simulink model "gluehofen"  (Simulink 3.00)
settings: Solver=ode45  StartTime=0.0  StopTime=80000  RelTol=1e-3
undefined symbols (not defined in the file): T

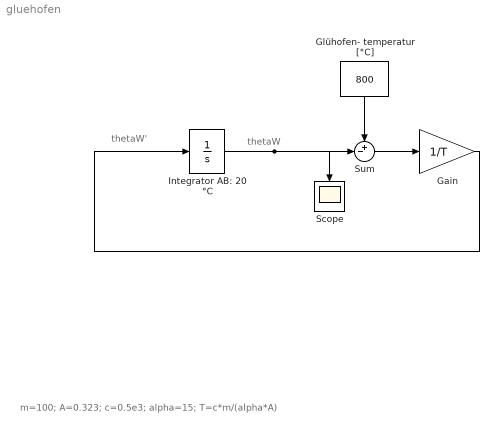
== system gluehofen ==
  note: m=100;
      | A=0.323;
      | c=0.5e3;
      | alpha=15;
      | T=c*m/(alpha*A)
  note: thetaW
  note: thetaW'
  Gain : Gain  Gain=1/T  SaturateOnIntegerOverflow=on
  Glühofen- temperatur [°C] : Constant  Orientation=down  Value=800
  Integrator AB: 20 °C : Integrator  ExternalReset=none  InitialConditionSource=internal  InitialCondition=20  LimitOutput=off  UpperSaturationLimit=inf  LowerSaturationLimit=-inf  ShowSaturationPort=off  ShowStatePort=off  AbsoluteTolerance=auto
  Scope : Scope
      settings: Orientation=down  TimeRange=auto  YMin=-5  YMax=5  SaveName=theta  DataFormat=Matrix
  Sum : Sum  Inputs=+-|  SaturateOnIntegerOverflow=on
  wires:
  Glühofen- temperatur [°C]/1 -> Sum/1
  Sum/1 -> Gain/1
  Gain/1 -> Integrator AB: 20 °C/1
  Integrator AB: 20 °C/1 -> Sum/2, Scope/1
